simulink model "p1"  (R2021b)
settings: Solver=VariableStepAuto  StartTime=0.0  StopTime=simTime  RelTol=1e-3
values from neighbouring files (symbols this model uses):
  ipMag = pi/4    (= 0.785398163397)    [p1.m]
  K = student_num(3)/5    [p1.m]
  ZOH = 1/50    (= 0.02)    [p1.m]
undefined symbols (not defined in the file or in its folder): denGamp, denGmot, numGamp, numGmot
settings Model: Creator=andre  LastModifiedBy=andre

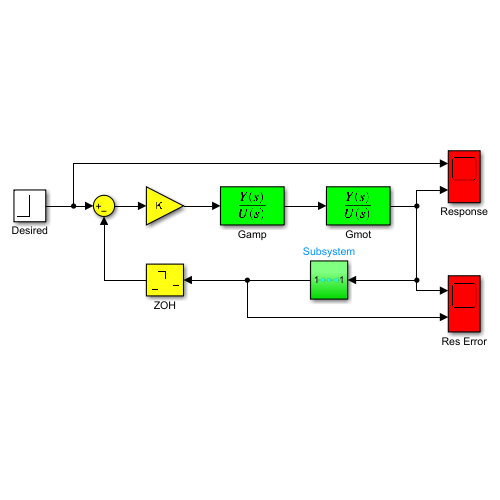
[thumbnail: Simulink's stored preview of the top-level diagram]
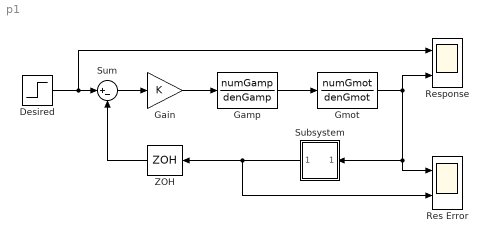
== system p1 ==
  Desired : Step  Time=0  After=ipMag  SampleTime=0
  Gain : Gain  Gain=K
  Gamp : TransferFcn  Numerator=numGamp  Denominator=denGamp
  Gmot : TransferFcn  Numerator=numGmot  Denominator=denGmot
  Res Error : Scope  NumInputPorts=2
  Response : Scope  NumInputPorts=2
  Subsystem : Subsystem
  Sum : Sum  Inputs=|+-
  ZOH : ZeroOrderHold  SampleTime=ZOH
  wires:
  Gmot/1 -> Response/2, Res Error/1, Subsystem/1(In1)
  Desired/1 -> Response/1, Sum/1
  ZOH/1 -> Sum/2
  Sum/1 -> Gain/1
  Gain/1 -> Gamp/1
  Gamp/1 -> Gmot/1
  Subsystem/1(Out1) -> Res Error/2, ZOH/1

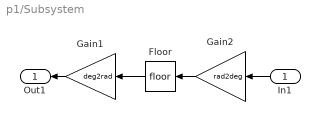
== system p1/Subsystem ==
  In1 : Inport
  Floor : Rounding
  Gain1 : Gain  Gain=deg2rad
  Gain2 : Gain  Gain=rad2deg
  Out1 : Outport
  wires:
  Floor/1 -> Gain1/1
  Gain2/1 -> Floor/1
  Gain1/1 -> Out1/1
  In1/1 -> Gain2/1
